simulink model "matlabprob5"  (R2020a)
settings: Solver=VariableStepAuto  StartTime=0.0  StopTime=10.0  RelTol=1e-3
libraries: simulink x2
settings Model: Creator=deepa  LastModifiedBy=deepa

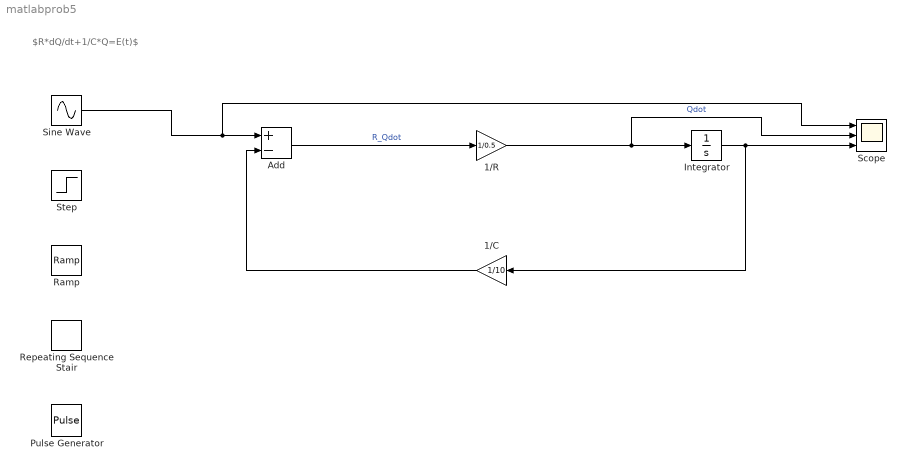
== system matlabprob5 ==
  note: $R*dQ/dt+1/C*Q=E(t)$
  1/C : Gain  Gain=1/10
  1/R : Gain  Gain=1/0.5
  Add : Sum  Inputs=+-
  Integrator : Integrator
  Pulse Generator : DiscretePulseGenerator  PulseType=Time based  Period=10  PulseWidth=5
  Ramp : simulink/Sources/Ramp  slope=1  start=0  InitialOutput=0
  Repeating Sequence Stair : simulink/Sources/Repeating Sequence Stair  OutValues=[3 1 4 2 1].'  tsamp=-1  OutMin=[]  OutMax=[]  OutDataTypeStr=double  OutputDataTypeScalingMode=double  OutDataType=fixdt(0,8)  ConRadixGroup=Best Precision: Vector-wise  OutScaling=2^-12
  Scope : Scope  NumInputPorts=3
  Sine Wave : Sin  SampleTime=0
  Step : Step  SampleTime=0
  wires:
  Add/1 -> 1/R/1  "R_Qdot"
  1/R/1 -> Scope/2, Integrator/1  "Qdot"
  Integrator/1 -> 1/C/1, Scope/3
  1/C/1 -> Add/2
  Sine Wave/1 -> Scope/1, Add/1
